simulink model "stellaris_test_adc_xpc"  (R2013a)
settings: Solver=FixedStepDiscrete  SolverMode=SingleTasking  StartTime=0.0  StopTime=inf  FixedStep=Ts  RelTol=1e-3
undefined symbols (not defined in the file or in its folder): Ts
libraries: speedgoatlib_IO101 x3, xpclib x1
settings Model: BufferReuse=off  Creator=peselnikmg  LastModifiedBy=peselnikmg
settings DataIOCC: SignalLoggingSaveFormat=ModelDataLogs
settings OptimizationCC: BlockReduction=off  BooleanDataType=off  OptimizeBlockIOStorage=off  BufferReuse=off  ExpressionFolding=off  ExpressionDepthLimit=2147483647  FoldNonRolledExpr=off  LocalBlockOutputs=off  InitFltsAndDblsToZero=on
settings DebuggingCC: SaveWithParameterizedLinksMsg=none  SignalResolutionControl=TryResolveAllWithWarning  MultiTaskDSMMsg=warning  FcnCallInpInsideContextMsg=UseLocalSettings  StrictBusMsg=None
settings HardwareCC: ProdIntDivRoundTo=Zero  ProdEndianess=LittleEndian  ProdHWDeviceType=Generic->32-bit x86 compatible
settings RTWCC: SystemTargetFile=xpctarget.tlc  TemplateMakefile=xpc_default_tmf  Description=xPC Target  ProcessScript=xpctarget_make_rtw_hook  RTWCompilerOptimization=On
settings xpcTargetCC: TargetFcnLib=ansi_tfl_tmw.mat  CodeReplacementLibrary=XPC_BLAS  ParMdlRefBuildCompliant=on  ConcurrentExecutionCompliant=on  CombineSignalStateStructs=off  MATLABClassNameForMDSCustomization=xpcAperiodicCustomization  GRTInterface=on  GenerateAllocFcn=off  xPCTaskExecutionProfile=off  xPCRL32EventNumber=5000  xPCLoadParamSetFile=off  xPCConcurrentTasks=off  xPCEnableSFAnimation=off

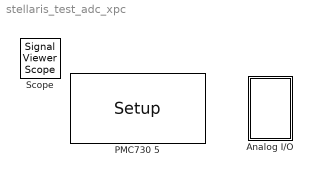
== system stellaris_test_adc_xpc ==
  Analog I/O : Subsystem
  PMC730 5 : speedgoatlib_IO101/Setup  group=Digital setup lower channel  id=1  pciSlot=-1  adStartChannel=1  adNumChannel=32  adCoupling=Single-ended  adRange=-10 .. 10 Volts  adAcqMode=Standard  daChannel=[1:8]  daReset=[1]  daInitValue=[0]  lowerChannel=[1:8]  lowerDirection=Input  lowerDIDebounce=0  lowerDOReset=[1]  lowerDOInitValues=[0]  upperChannel=[1:8]  upperDirection=Output  upperDIDebounce=0  upperDOReset=0  upperDOInitValues=0
  Scope : SignalViewerScope  IOType=viewer  ZoomMode=xonly  RefreshTime=0.035000

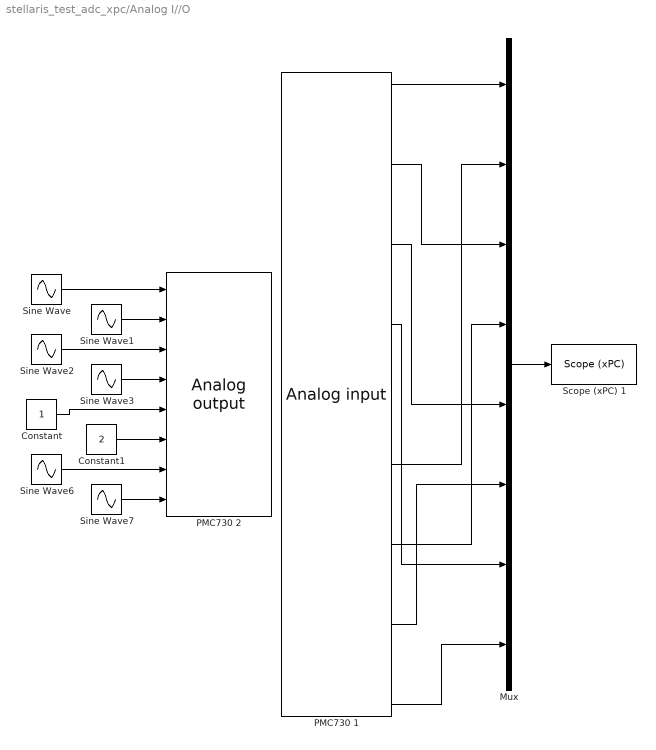
== system stellaris_test_adc_xpc/Analog I//O ==
  Constant : Constant
  Constant1 : Constant  Value=2
  Mux : Mux  Inputs=8
  PMC730 1 : speedgoatlib_IO101/Analog input  id=1  startChannel=1  numChannels=32  coupling=2  range=3  acqMode=1  outpMode=Values  ts=Ts  pciSlot=-1
  PMC730 2 : speedgoatlib_IO101/Analog output  id=1  channel=[1,2,3,4,5,6,7,8]  reset=[1,1,1,1,1,1,1,1]  initValue=[0,0,0,0,0,0,0,0]  ts=Ts  pciSlot=-1
  Scope (xPC) 1 : xpclib/Misc./Scope (xPC)   scopeno=2  scopetype=Target  autostart=on  viewmode=Graphical redraw  formatstr='%15.6f'  grid=on  ylimits=[0,0]  nosamples=250  noprepostsamples=0  interleave=1  triggermode=Signal triggering  triggersignal=1  trigsignalfromport=off  triggerlevel=0.0  triggerslope=Rising  triggerscope=1  triggersample=0  filename=data.dat  mode=Lazy  writesize=512  autorestart=off  dynamicfilemode=off  maxwritefilesize=512*1024^2
  Sine Wave : Sin  Frequency=2*pi*1/Ts/50  SampleTime=Ts
  Sine Wave1 : Sin  Amplitude=2  Frequency=2*pi*1/Ts/50  SampleTime=Ts
  Sine Wave2 : Sin  Amplitude=3  Frequency=2*pi*1/Ts/50  SampleTime=Ts
  Sine Wave3 : Sin  Amplitude=4  Frequency=2*pi*1/Ts/50  SampleTime=Ts
  Sine Wave6 : Sin  Amplitude=1.5  Bias=1.5  Frequency=2*pi*1/Ts/500  SampleTime=Ts
  Sine Wave7 : Sin  Amplitude=8  Frequency=2*pi*1/Ts/50  SampleTime=Ts
  wires:
  PMC730 1/32 -> Mux/8
  PMC730 1/13 -> Mux/7
  PMC730 1/28 -> Mux/6
  PMC730 1/9 -> Mux/5
  PMC730 1/24 -> Mux/4
  PMC730 1/5 -> Mux/3
  PMC730 1/20 -> Mux/2
  PMC730 1/1 -> Mux/1
  Sine Wave6/1 -> PMC730 2/7
  Constant1/1 -> PMC730 2/6
  Constant/1 -> PMC730 2/5
  Sine Wave3/1 -> PMC730 2/4
  Sine Wave2/1 -> PMC730 2/3
  Sine Wave1/1 -> PMC730 2/2
  Sine Wave/1 -> PMC730 2/1
  Sine Wave7/1 -> PMC730 2/8
  Mux/1 -> Scope (xPC) 1/1
